simulink model "HalfCar_BodyModel"  (R2018b)
settings: Solver=VariableStepAuto  StartTime=0.0  StopTime=5  RelTol=1e-3
values from neighbouring files (symbols this model uses):
  a = 1.25    [SetCoefficients.m]    (also in SetCoefficients_HC.m)
  b = 1.4    [SetCoefficients.m]    (also in SetCoefficients_HC.m)
  g = 9.81    [SetCoefficients.m]    (also in SetCoefficients_HC.m)
  I = 600    [SetCoefficients.m]    (also in SetCoefficients_HC.m)
  mb = 500    [SetCoefficients.m]    (also in SetCoefficients_HC.m)
settings Model: Creator=joebe  LastModifiedBy=joebe

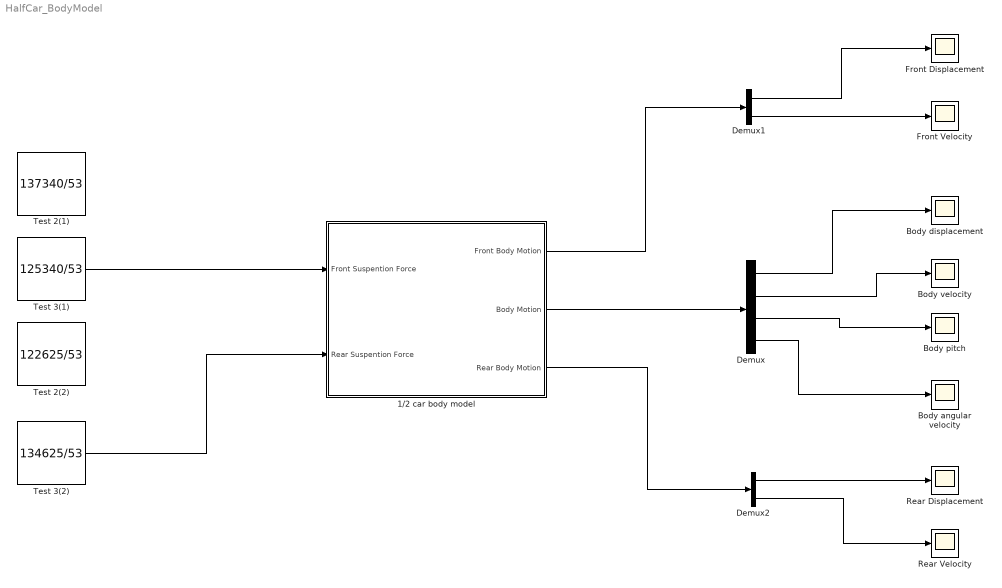
== system HalfCar_BodyModel ==
  1/2 car body model : Subsystem
  Body angular velocity : Scope
  Body displacement : Scope
  Body pitch : Scope
  Body velocity : Scope
  Demux : Demux
  Demux1 : Demux  Outputs=2
  Demux2 : Demux  Outputs=2
  Front Displacement : Scope
  Front Velocity : Scope
  Rear Displacement : Scope
  Rear Velocity : Scope
  Test 2(1) : Constant  Value=137340/53
  Test 2(2) : Constant  Value=122625/53
  Test 3(1) : Constant  Value=125340/53
  Test 3(2) : Constant  Value=134625/53
  wires:
  1/2 car body model/2(Body Motion) -> Demux/1
  Demux/1 -> Body displacement/1
  Demux/2 -> Body velocity/1
  Demux/3 -> Body pitch/1
  Demux/4 -> Body angular velocity/1
  1/2 car body model/3(Rear Body Motion) -> Demux2/1
  1/2 car body model/1(Front Body Motion) -> Demux1/1
  Demux1/2 -> Front Velocity/1
  Demux1/1 -> Front Displacement/1
  Demux2/1 -> Rear Displacement/1
  Demux2/2 -> Rear Velocity/1
  Test 3(1)/1 -> 1/2 car body model/1(Front Suspention Force)
  Test 3(2)/1 -> 1/2 car body model/2(Rear Suspention Force)

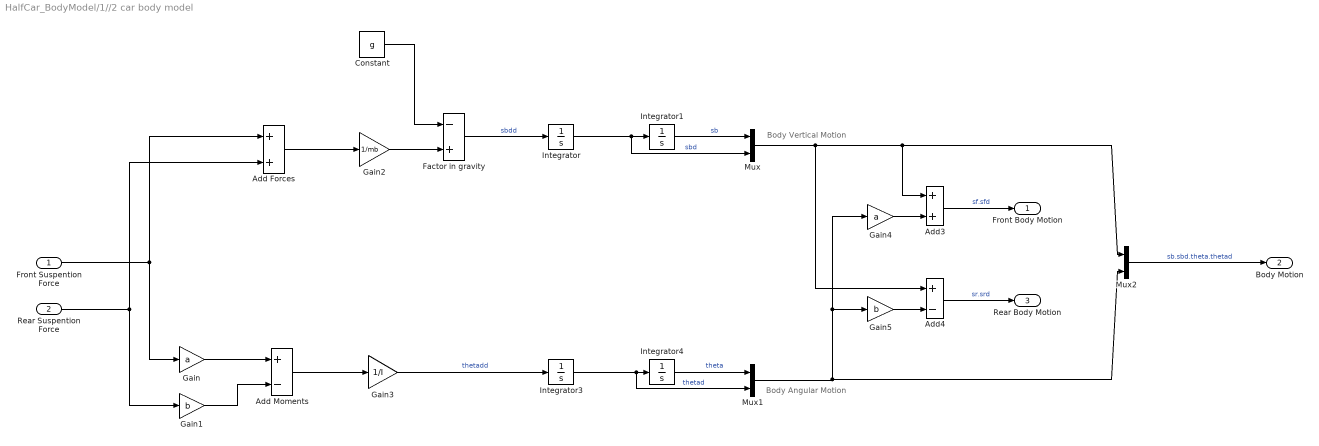
== system HalfCar_BodyModel/1//2 car body model ==
  note: Body Angular Motion
  note: Body Vertical Motion
  Front Suspention Force : Inport
  Rear Suspention Force : Inport  Port=2
  Add Forces : Sum
  Add Moments : Sum  Inputs=+-
  Add3 : Sum
  Add4 : Sum  Inputs=+-
  Constant : Constant  Value=g
  Factor in gravity : Sum  Inputs=-+
  Gain : Gain  Gain=a
  Gain1 : Gain  Gain=b
  Gain2 : Gain  Gain=1/mb
  Gain3 : Gain  Gain=1/I
  Gain4 : Gain  Gain=a
  Gain5 : Gain  Gain=b
  Integrator{,1,3..4} (4 alike) : Integrator
  Mux : Mux  Inputs=2
  Mux1 : Mux  Inputs=2
  Mux2 : Mux  Inputs=2
  Front Body Motion : Outport
  Body Motion : Outport  Port=2
  Rear Body Motion : Outport  Port=3
  wires:
  Add Forces/1 -> Gain2/1
  Mux1/1 -> Gain4/1, Gain5/1, Mux2/2
  Integrator3/1 -> Mux1/2, Integrator4/1  "thetad"
  Add Moments/1 -> Gain3/1
  Gain3/1 -> Integrator3/1  "thetadd"
  Mux2/1 -> Body Motion/1  "sb.sbd.theta.thetad"
  Gain2/1 -> Factor in gravity/2
  Mux/1 -> Add4/1, Add3/1, Mux2/1
  Gain4/1 -> Add3/2
  Gain/1 -> Add Moments/1
  Integrator4/1 -> Mux1/1  "theta"
  Integrator/1 -> Mux/2, Integrator1/1  "sbd"
  Rear Suspention Force/1 -> Add Forces/2, Gain1/1
  Front Suspention Force/1 -> Gain/1, Add Forces/1
  Integrator1/1 -> Mux/1  "sb"
  Gain1/1 -> Add Moments/2
  Add3/1 -> Front Body Motion/1  "sf.sfd"
  Gain5/1 -> Add4/2
  Constant/1 -> Factor in gravity/1
  Factor in gravity/1 -> Integrator/1  "sbdd"
  Add4/1 -> Rear Body Motion/1  "sr.srd"
